simulink model "B_Comp"  (R2024b)
settings: Solver=ode23tb  StartTime=0.0  StopTime=8000  RelTol=1e-3
PreLoadFcn:
  | Load_Maps
InitFcn:
  | B_init_compressor
StopFcn:
  | plotmap
libraries: simulink_extras x5, slpidlib x2, simulink x2
settings Model: Creator=aa921  LastModifiedBy=mmercang
settings DataIOCC: FinalStateName=xfinal  InitialState=x_comp  LoadInitialState=on  SaveFinalState=on  SaveFormat=Structure  SaveState=on  ReturnWorkspaceOutputsName=out_comp

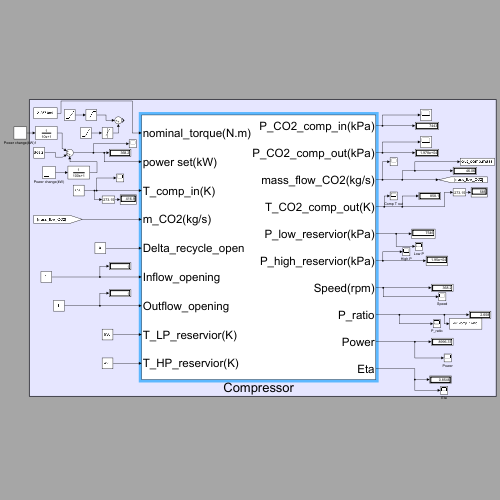
[thumbnail: Simulink's stored preview of the top-level diagram]
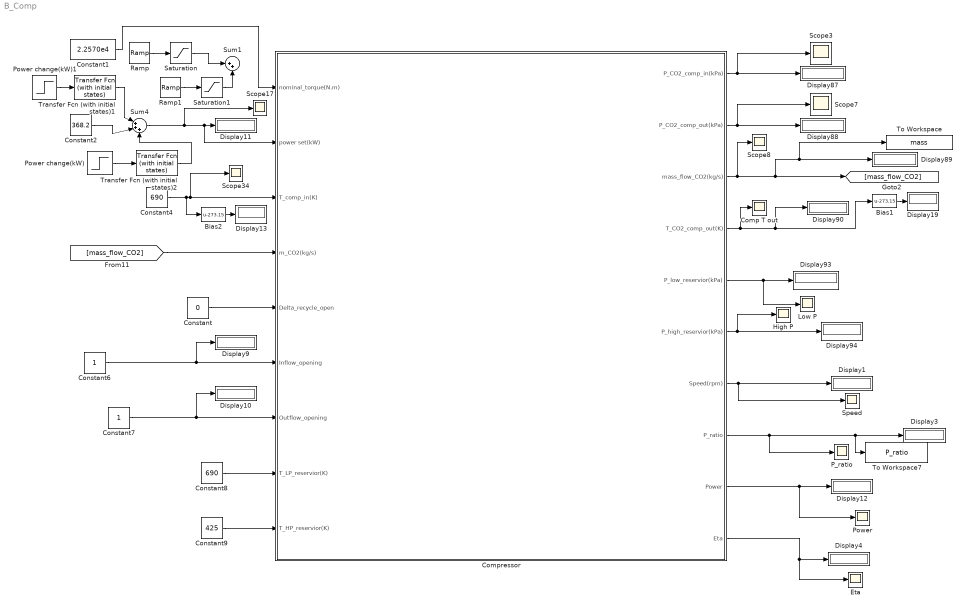
== system B_Comp ==
  Bias1 : Bias  Bias=-273.15  SaturateOnIntegerOverflow=off
  Bias2 : Bias  Bias=-273.15  SaturateOnIntegerOverflow=off
  Comp T out : Scope
  Compressor : Subsystem
  Constant : Constant  Value=0
  Constant1 : Constant  Value=2.2570e4
  Constant2 : Constant  Value=368.2
  Constant4 : Constant  Value=690
  Constant6 : Constant
  Constant7 : Constant
  Constant8 : Constant  Value=690
  Constant9 : Constant  Value=425
  Display{1,3..4,9..13,19,87..90,93..94} (15 alike) : Display
      Display12 settings: Format=bank
  Eta : Scope
  High P : Scope
  Low P : Scope
  P_ratio : Scope
  Power : Scope
  Power change(kW) : Step  Time=3000  After=368.2  SampleTime=0
  Power change(kW)1 : Step  Time=1500  After=-368.2  SampleTime=0
  Ramp : simulink/Sources/Ramp  slope=-50  start=1000  InitialOutput=2.2570e4
  Ramp1 : simulink/Sources/Ramp  slope=50  start=3000  InitialOutput=0
  Saturation : Saturate  UpperLimit=2.2570e4  LowerLimit=0
  Saturation1 : Saturate  UpperLimit=2.2570e4  LowerLimit=0
  Scope{3,7..8,17,34} (5 alike) : Scope
  Speed : Scope
  Sum1 : Sum  Inputs=|++
  Sum4 : Sum  Inputs=|+++
  To Workspace : ToWorkspace  VariableName=mass  SampleTime=-1
      settings: Save2DSignal=2-D array (concatenate along first dimension)
  To Workspace7 : ToWorkspace  VariableName=P_ratio  SampleTime=-1
      settings: Save2DSignal=2-D array (concatenate along first dimension)
  Transfer Fcn (with initial states)1 : simulink_extras/Additional Linear/Transfer Fcn (with initial states)  N=[1]  D="[10  1]"  X0=0
  Transfer Fcn (with initial states)2 : simulink_extras/Additional Linear/Transfer Fcn (with initial states)  N=[1]  D="[100  1]"  X0=0
  wires:
  Compressor/1(P_CO2_comp_in(kPa)) -> Scope3/1, Display87/1
  Compressor/7(Speed(rpm)) -> Speed/1, Display1/1
  Constant7/1 -> Display10/1, Compressor/7(Outflow_opening)
  Constant8/1 -> Compressor/8(T_LP_reservior(K))
  Constant2/1 -> Sum4/2
  [mass_flow_CO2] -> Compressor/4(m_CO2(kg/s))
  Constant/1 -> Compressor/5(Delta_recycle_open)
  Constant4/1 -> Scope34/1, Compressor/3(T_comp_in(K)), Bias2/1
  Compressor/6(P_high_reservior(kPa)) -> Display94/1, High P/1
  Compressor/5(P_low_reservior(kPa)) -> Low P/1, Display93/1
  Sum4/1 -> Compressor/2(power set(kW)), Display11/1, Scope17/1
  Constant6/1 -> Display9/1, Compressor/6(Inflow_opening)
  Compressor/4(T_CO2_comp_out(K)) -> Bias1/1, Display90/1, Comp T out/1
  Bias2/1 -> Display13/1
  Constant9/1 -> Compressor/9(T_HP_reservior(K))
  Bias1/1 -> Display19/1
  Power change(kW)/1 -> Transfer Fcn (with initial states)2/1
  Compressor/9(Power) -> Display12/1, Power/1
  Compressor/10(Eta) -> Display4/1, Eta/1
  Compressor/2(P_CO2_comp_out(kPa)) -> Display88/1, Scope7/1
  Compressor/3(mass_flow_CO2(kg/s)) -> [mass_flow_CO2], To Workspace/1, Display89/1, Scope8/1
  Compressor/8(P_ratio) -> To Workspace7/1, Display3/1, P_ratio/1
  Ramp/1 -> Saturation/1
  Saturation/1 -> Sum1/1
  Power change(kW)1/1 -> Transfer Fcn (with initial states)1/1
  Ramp1/1 -> Saturation1/1
  Saturation1/1 -> Sum1/2
  Constant1/1 -> Compressor/1(nominal_torque(N.m))
  Transfer Fcn (with initial states)1/1 -> Sum4/1
  Transfer Fcn (with initial states)2/1 -> Sum4/3

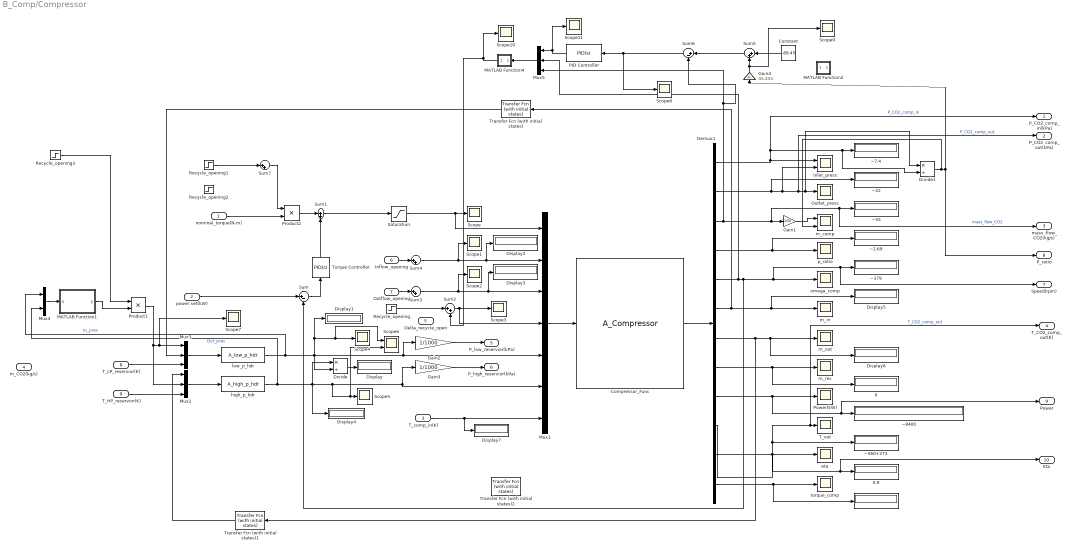
== system B_Comp/Compressor ==
  nominal_torque(N.m) : Inport
  power set(kW) : Inport  Port=2
  T_comp_in(K) : Inport  Port=3
  m_CO2(kg/s) : Inport  Port=4
  Delta_recycle_open : Inport  Port=5
  Inflow_opening : Inport  Port=6
  Outflow_opening : Inport  Port=7
  T_LP_reservior(K) : Inport  Port=8
  T_HP_reservior(K) : Inport  Port=9
  " " : Display
  0 : Display
  0.9 : Display
  Compressor_Func : S-Function  FunctionName=A_Compressor  Parameters=Param_COMP  SFunctionDeploymentMode=off  EnableBusSupport=off
  Constant : Constant  Value=-89.45
  Demux1 : Demux  Outputs=12
  Display{,1..7} (8 alike) : Display
  Divide : Product  Inputs=*/
  Divide1 : Product  Inputs=*/
  Gain1 : Gain  Gain=1/50
  Gain2 : Gain  Gain=1/1000
  Gain3 : Gain  Gain=1/1000
  Gain4 : Gain  Gain=45.455
  Inlet_press : Scope  NumInputPorts=2
  MATLAB Function1 : MATLAB Function  TreatAsAtomicUnit=on
  MATLAB Function2 : MATLAB Function  TreatAsAtomicUnit=on
  MATLAB Function4 : MATLAB Function  TreatAsAtomicUnit=on
  Mux1 : Mux  Inputs=7
  Mux2 : Mux  Inputs=3
  Mux3 : Mux  Inputs=3
  Mux4 : Mux  Inputs=2
  Mux5 : Mux  Inputs=3
  Outlet_press : Scope
  PID Controller : slpidlib/PID Controller  Controller=PID  Form=Parallel  TimeDomain=Continuous-time  UseExternalTs=off  SampleTime=-1  IntegratorMethod=Forward Euler  FilterMethod=Forward Euler  ControllerParametersSource=internal  P=0.01  I=0.001  UseKiTs=off  D=0  UseExternalDerivativeSource=off  N=100  UseFilter=on  TunerSelectOption=Transfer Function Based (PID Tuner App)  InitialConditionSource=internal  InitialConditionForIntegrator=0  InitialConditionForFilter=0  DifferentiatorICPrevScaledInput=0  ExternalReset=none  TrackingMode=off  Kt=1  LimitOutput=on  SatLimitsSource=internal  UpperSaturationLimit=1  LowerSaturationLimit=0  LinearizeAsGain=on  AntiWindupMode=back-calculation  Kb=1  LimitIntegrator=on  UpperIntegratorSaturationLimit=inf  LowerIntegratorSaturationLimit=-inf  POutMin=[]  POutMax=[]  IOutMin=[]  IOutMax=[]  DOutMin=[]  DOutMax=[]  NOutMin=[]  NOutMax=[]  SumOutMin=[]  SumOutMax=[]  SaturationOutMin=[]  SaturationOutMax=[]  PParamMin=[]  PParamMax=[]  IParamMin=[]  IParamMax=[]  DParamMin=[]  DParamMax=[]  NParamMin=[]  NParamMax=[]  KbParamMin=[]  KbParamMax=[]  KtParamMin=[]  KtParamMax=[]  KbOutMin=[]  KbOutMax=[]  KtOutMin=[]  KtOutMax=[]  IntegratorOutMin=[]  IntegratorOutMax=[]  FilterOutMin=[]  FilterOutMax=[]  SumI1OutMin=[]  SumI1OutMax=[]  SumI2OutMin=[]  SumI2OutMax=[]  SumI3OutMin=[]  SumI3OutMax=[]  SumI4OutMin=[]  SumI4OutMax=[]  SumDOutMin=[]  SumDOutMax=[]  DifferentiatorOutMin=[]  DifferentiatorOutMax=[]  FilterDiffOutCoefMin=[]  FilterDiffOutCoefMax=[]  ReciprocalOutMin=[]  ReciprocalOutMax=[]  SumDenOutMin=[]  SumDenOutMax=[]  SumNumOutMin=[]  SumNumOutMax=[]  DivideOutMin=[]  DivideOutMax=[]  UdiffTsProdOutMin=[]  UdiffTsProdOutMax=[]  NTsProdOutMin=[]  NTsProdOutMax=[]  UintegralTsProdOutMin=[]  UintegralTsProdOutMax=[]  UngainTsProdOutMin=[]  UngainTsProdOutMax=[]  ClampingZeroOutDataTypeStr=Inherit: Inherit via back propagation  ClampingZeroOutMin=[]  ClampingZeroOutMax=[]  FilterDenConstantOutDataTypeStr=Inherit: Inherit via back propagation  FilterDenConstantOutMin=[]  FilterDenConstantOutMax=[]  PCopyOutDataTypeStr=Inherit: Inherit via back propagation  PCopyOutMin=[]  PCopyOutMax=[]  NCopyOutDataTypeStr=Inherit: Inherit via back propagation  NCopyOutMin=[]  NCopyOutMax=[]  IntegratorContinuousStateAttributes=''  IntegratorStateMustResolveToSignalObject=off  IntegratorRTWStateStorageClass=Auto  FilterContinuousStateAttributes=''  FilterStateMustResolveToSignalObject=off  FilterRTWStateStorageClass=Auto  ParallelPVariant=InternalParameters  IdealPVariant=Disabled  IVariant=InternalParameters  DVariant=InternalParameters  IntegratorVariant=Continuous  SatVariant=Enabled  AWVariant=BackCalculation  PCopyVariant=Disabled  TRVariant=Disabled  FdbkBlocksVariant=Forward  IdealPFdbkVariant=Disabled  SatFdbkVariant=Disabled  DerivativeFilterVariant=ContFilter  NVariant=InternalParameters  NCopyVariant=Disabled  FilterICVariant=InternalICsFilter  IntegratorICVariant=InternalICs  ExternalResetVariant=Disabled  TRSumVariant=Passthrough  SumFdbkVariant=Disabled  SumVariant=Sum_PID  TsampFilterVariant=InternalTs  TsampNgainVariant=Passthrough  TsampIntegralVariant=Disabled_SignalSpec  ExternalSaturationOutDataTypeStr=Inherit: Same as second input  DerivativeSourceVariant=ErrorSignal  PreIntVariant=InternalPreInt
  Power(kW) : Scope
  Product1 : Product
  Product2 : Product
  Recycle_opening : Step  Time=2005  After=0  SampleTime=0
  Recycle_opening1 : Step  Time=2000  Before=1  SampleTime=0
  Recycle_opening2 : Step  Time=3500  SampleTime=0
  Recycle_opening3 : Step  Time=2000  Before=1  SampleTime=0
  Saturation : Saturate  UpperLimit=2.2570e4  LowerLimit=0
  Scope{,1..5,7..11} (11 alike) : Scope
  Scope6 : Scope  NumInputPorts=2
  Sum : Sum  Inputs=|+-
  Sum{1..5,7} (6 alike) : Sum  Inputs=|++
  Sum6 : Sum  Inputs=|+-
  T_out : Scope
  Torque Controller : slpidlib/PID Controller  Controller=PID  Form=Parallel  TimeDomain=Continuous-time  UseExternalTs=off  SampleTime=-1  IntegratorMethod=Forward Euler  FilterMethod=Forward Euler  ControllerParametersSource=internal  P=200  I=10  UseKiTs=off  D=0  UseExternalDerivativeSource=off  N=100  UseFilter=on  TunerSelectOption=Transfer Function Based (PID Tuner App)  InitialConditionSource=internal  InitialConditionForIntegrator=0  InitialConditionForFilter=0  DifferentiatorICPrevScaledInput=0  ExternalReset=none  TrackingMode=off  Kt=1  LimitOutput=off  SatLimitsSource=internal  UpperSaturationLimit=inf  LowerSaturationLimit=-inf  LinearizeAsGain=on  AntiWindupMode=none  Kb=1  LimitIntegrator=off  UpperIntegratorSaturationLimit=inf  LowerIntegratorSaturationLimit=-inf  POutMin=[]  POutMax=[]  IOutMin=[]  IOutMax=[]  DOutMin=[]  DOutMax=[]  NOutMin=[]  NOutMax=[]  SumOutMin=[]  SumOutMax=[]  SaturationOutMin=[]  SaturationOutMax=[]  PParamMin=[]  PParamMax=[]  IParamMin=[]  IParamMax=[]  DParamMin=[]  DParamMax=[]  NParamMin=[]  NParamMax=[]  KbParamMin=[]  KbParamMax=[]  KtParamMin=[]  KtParamMax=[]  KbOutMin=[]  KbOutMax=[]  KtOutMin=[]  KtOutMax=[]  IntegratorOutMin=[]  IntegratorOutMax=[]  FilterOutMin=[]  FilterOutMax=[]  SumI1OutMin=[]  SumI1OutMax=[]  SumI2OutMin=[]  SumI2OutMax=[]  SumI3OutMin=[]  SumI3OutMax=[]  SumI4OutMin=[]  SumI4OutMax=[]  SumDOutMin=[]  SumDOutMax=[]  DifferentiatorOutMin=[]  DifferentiatorOutMax=[]  FilterDiffOutCoefMin=[]  FilterDiffOutCoefMax=[]  ReciprocalOutMin=[]  ReciprocalOutMax=[]  SumDenOutMin=[]  SumDenOutMax=[]  SumNumOutMin=[]  SumNumOutMax=[]  DivideOutMin=[]  DivideOutMax=[]  UdiffTsProdOutMin=[]  UdiffTsProdOutMax=[]  NTsProdOutMin=[]  NTsProdOutMax=[]  UintegralTsProdOutMin=[]  UintegralTsProdOutMax=[]  UngainTsProdOutMin=[]  UngainTsProdOutMax=[]  ClampingZeroOutDataTypeStr=Inherit: Inherit via back propagation  ClampingZeroOutMin=[]  ClampingZeroOutMax=[]  FilterDenConstantOutDataTypeStr=Inherit: Inherit via back propagation  FilterDenConstantOutMin=[]  FilterDenConstantOutMax=[]  PCopyOutDataTypeStr=Inherit: Inherit via back propagation  PCopyOutMin=[]  PCopyOutMax=[]  NCopyOutDataTypeStr=Inherit: Inherit via back propagation  NCopyOutMin=[]  NCopyOutMax=[]  IntegratorContinuousStateAttributes=''  IntegratorStateMustResolveToSignalObject=off  IntegratorRTWStateStorageClass=Auto  FilterContinuousStateAttributes=''  FilterStateMustResolveToSignalObject=off  FilterRTWStateStorageClass=Auto  ParallelPVariant=InternalParameters  IdealPVariant=Disabled  IVariant=InternalParameters  DVariant=InternalParameters  IntegratorVariant=Continuous  SatVariant=Disabled  AWVariant=Passthrough  PCopyVariant=Disabled  TRVariant=Disabled  FdbkBlocksVariant=Forward  IdealPFdbkVariant=Disabled  SatFdbkVariant=Disabled  DerivativeFilterVariant=ContFilter  NVariant=InternalParameters  NCopyVariant=Disabled  FilterICVariant=InternalICsFilter  IntegratorICVariant=InternalICs  ExternalResetVariant=Disabled  TRSumVariant=Passthrough  SumFdbkVariant=Disabled  SumVariant=Sum_PID  TsampFilterVariant=InternalTs  TsampNgainVariant=Passthrough  TsampIntegralVariant=Disabled_SignalSpec  ExternalSaturationOutDataTypeStr=Inherit: Same as second input  DerivativeSourceVariant=ErrorSignal  PreIntVariant=InternalPreInt
  Transfer Fcn (with initial states) : simulink_extras/Additional Linear/Transfer Fcn (with initial states)  N=[1]  D="[1  1]"  X0=53.0908043651412
  Transfer Fcn (with initial states)1 : simulink_extras/Additional Linear/Transfer Fcn (with initial states)  N=[1]  D="[1  1]"  X0=53.0908043651412
  Transfer Fcn (with initial states)2 : simulink_extras/Additional Linear/Transfer Fcn (with initial states)  N=[1]  D="[1  1]"  X0=8730.07996310326
  eta : Scope
  high_p_hdr : S-Function  FunctionName=A_high_p_hdr  Parameters=Param_COMP  SFunctionDeploymentMode=off  EnableBusSupport=off
  low_p_hdr : S-Function  FunctionName=A_low_p_hdr  Parameters=Param_COMP  SFunctionDeploymentMode=off  EnableBusSupport=off
  m_comp : Scope  NumInputPorts=2
  m_in : Scope
  m_out : Scope
  m_rec : Scope
  omega_comp : Scope
  p_ratio : Scope
  torque_comp : Scope
  ~2.69 : Display
  ~{22,55,379,8400} (4 alike) : Display
      ~8400 settings: Format=long_e
  ~560+273 : Display
  ~7.4 : Display
  P_CO2_comp_in(kPa) : Outport
  P_CO2_comp_out(kPa) : Outport  Port=2
  mass_flow_CO2(kg/s) : Outport  Port=3
  T_CO2_comp_out(K) : Outport  Port=4
  P_low_reservior(kPa) : Outport  Port=5
  P_high_reservior(kPa) : Outport  Port=6
  Speed(rpm) : Outport  Port=7
  P_ratio : Outport  Port=8
  Power : Outport  Port=9
  Eta : Outport  Port=10
  wires:
  Demux1/10 -> T_CO2_comp_out(K)/1, T_out/1, ~560+273/1  "T_CO2_comp_out"
  Demux1/12 -> " "/1, torque_comp/1
  Demux1/6 -> Transfer Fcn (with initial states)/1, m_in/1, Display5/1
  Demux1/3 -> Mux5/3, Sum6/2, ~55/1, mass_flow_CO2(kg/s)/1, Gain1/1  "mass_flow_CO2"
  low_p_hdr/1 -> Mux4/1, Gain2/1, Mux1/5, Divide/2, Display1/1, Scope6/1, Scope4/1  "In_pres"
  Demux1/2 -> Inlet_press/2, P_CO2_comp_out(kPa)/1, Divide1/1, Outlet_press/1, ~22/1  "P_CO2_comp_out"
  Compressor_Func/1 -> Demux1/1
  Demux1/8 -> m_rec/1, 0/1
  Demux1/1 -> Inlet_press/1, P_CO2_comp_in(kPa)/1, Divide1/2, ~7.4/1  "P_CO2_comp_in"
  Demux1/11 -> eta/1, Eta/1, 0.9/1
  Demux1/9 -> Power/1, ~8400/1, Power(kW)/1
  Sum/1 -> Torque Controller/1
  Mux1/1 -> Compressor_Func/1
  Divide/1 -> Display/1
  high_p_hdr/1 -> Mux4/2, Divide/1, Display4/1, Scope6/2, Scope5/1, Gain3/1, Mux1/6  "Out_pres"
  T_comp_in(K)/1 -> Display7/1, Mux1/7
  Mux3/1 -> low_p_hdr/1
  Mux2/1 -> high_p_hdr/1
  Demux1/5 -> Mux5/2, omega_comp/1, Speed(rpm)/1, ~379/1, Sum/2
  Transfer Fcn (with initial states)/1 -> Mux3/2
  Transfer Fcn (with initial states)1/1 -> Mux2/1
  Gain2/1 -> P_low_reservior(kPa)/1
  Gain3/1 -> P_high_reservior(kPa)/1
  Demux1/4 -> ~2.69/1, p_ratio/1
  Sum2/1 -> Scope3/1, Mux1/4
  Outflow_opening/1 -> Sum3/1
  Inflow_opening/1 -> Sum4/1
  Sum4/1 -> Scope1/1, Display2/1, Mux1/2
  Sum3/1 -> Scope2/1, Display3/1, Mux1/3
  Sum1/1 -> Saturation/1
  power set(kW)/1 -> Sum/1
  T_HP_reservior(K)/1 -> Mux2/3
  T_LP_reservior(K)/1 -> Mux3/3
  Constant/1 -> Sum5/1
  Sum5/1 -> Sum6/1
  Sum6/1 -> Scope8/1, PID Controller/1
  Demux1/7 -> Transfer Fcn (with initial states)1/1, m_out/1, Display6/1
  Mux4/1 -> MATLAB Function1/1(u)
  Product1/1 -> Scope7/1, Mux3/1, Mux2/2
  Recycle_opening3/1 -> Product1/1
  MATLAB Function1/1(y) -> Product1/2
  nominal_torque(N.m)/1 -> Product2/2
  Recycle_opening1/1 -> Sum7/1
  Sum7/1 -> Product2/1
  Product2/1 -> Sum1/1
  Gain1/1 -> m_comp/1
  Recycle_opening/1 -> Sum2/1
  Divide1/1 -> m_comp/2, Gain4/1, P_ratio/1
  Gain4/1 -> Scope9/1, Sum5/2
  PID Controller/1 -> Scope11/1, Mux5/1
  Mux5/1 -> MATLAB Function4/1(u)
  MATLAB Function4/1(y) -> Sum2/2, Scope10/1
  Torque Controller/1 -> Sum1/2
  Saturation/1 -> Mux1/1, Scope/1

== matlab function B_Comp/Compressor/MATLAB Function2 ==
  data: u input; y output
function y = fcn(u)

if u<5

y = -40;
else

y=u;
end

== matlab function B_Comp/Compressor/MATLAB Function4 ==
  data: u input; y output
function y = fcn(u)

if u(2)<180 && u(3)<30

y = 1;

else

y=u(1);
end

== matlab function B_Comp/Compressor/MATLAB Function1 ==
  data: u input; y output
function y = fcn(u)

Valve_in_gain=0.1071*1.34;
In_pres=u(1);
Out_pres=u(2);

m_in     = Valve_in_gain*46.0641/496.2541 * sqrt(abs(Out_pres - In_pres)) * (Out_pres - In_pres)/abs(Out_pres - In_pres);
y = m_in;
